simulink model "MPC_mobile_base_KIN_IPOPT_fast"  (R2018b)
settings: Solver=ode4  StartTime=0.0  StopTime=inf  FixedStep=Tsample  RelTol=1e-3
values from neighbouring files (symbols this model uses):
  N = 20    [STEP.m]    (also in ZZ_MIO_STEP.m = 8)
  T = 0.2    [STEP.m]    (also in ZZ_MIO_STEP.m)
  Tsample = 0.01    [STEP.m]    (also in ZZ_MIO_STEP.m)
  xd = [linspace(0,5,length(tt));0.5*ones(size(tt));zeros(size(tt))]    [STEP.m]    (also in ZZ_MIO_STEP.m = [linspace(0,5,length(tt));0.25*ones(size(tt));zeros(size(tt))
undefined symbols (not defined in the file or in its folder): DiscIntNeverNeededParam
libraries: simulink x2, templibrary x1
settings Model: Creator=francesco  LastModifiedBy=francesco

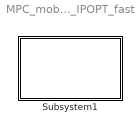
== system MPC_mobile_base_KIN_IPOPT_fast ==
  Subsystem1 : Subsystem  InitFcn=|
      | clearvars -EXCEPT  xd N T Tsample tt
      | 
      | import casadi.*
      | 
      | 
      | %%%%%%%%%%%% SETTINGS %%%%%%%%%%%%%%%%%%%%%
      | 
      | fs = 1/T; % Sampling frequency [hz]
      | m  = 2;
      | T_horizon=(0:N-1)*T;
      | 
      | Ak= diag([100    100    100]);
      | 
      | Vpmax=inf;  %  [m/s^2]
      | Wpmax=3; %  [rad/s^2]
      | 
      | Vpmax=Vpmax*T;
      | Wpmax=Wpmax*T;
      | %%%%%%%%%%%% MODELING %%%%%%%%%%%%%%%%%%%%%
      | x  = MX.sym('x',3);
      | Xd  = MX.sym('Xd',3,N);
      | t  = MX.sym('t');
      | x0 = MX.sym('x0',3);
      | U0  = MX.sym('U0',2,1);
      | 
      | p = MX.sym('p',8);
      | 
      | % xdot = [(p(1)*t^2+p(2)*t+p(3))*cos(x(3)); ...
      | %         (p(1)*t^2+p(2)*t+p(3))*sin(x(3)); ...
      | %         (p(4)*t^3+p(5)*t^2+p(6)*t+p(7))         ];
      | 
      | xdot = [(p(1)*t^3+p(2)*t^2+p(3)*t+p(4))*cos(x(3)); ...
      |         (p(1)*t^3+p(2)*t^2+p(3)*t+p(4))*sin(x(3)); ...
      |         (p(5)*t^3+p(6)*t^2+p(7)*t+p(8))         ];
      | 
      | % Form an ode function
      | ode = Function('ode',{x,p,t},{xdot});
      | 
      | %%%%%%%%%%%% Creating a simulator %%%%%%%%%%
      | N_steps_per_sample = 2;
      | dt = 1/fs/N_steps_per_sample;
      | 
      | % Build an integrator for this system: Runge Kutta 4 integrator
      | k1 = ode(x,p,t);
      | k2 = ode(x+dt/2.0*k1,p,t+dt/2.0);
      | k3 = ode(x+dt/2.0*k2,p,t+dt/2.0);
      | k4 = ode(x+dt*k3,p,t+dt/2.0);
      | 
      | xstep = x+dt/6.0*(k1+2*k2+2*k3+k4);
      | 
      | % Create a function that simulates one step propagation in a sample
      | one_step = Function('one_step',{x, p, t},{xstep});
      | 
      | X = x;
      | for i=1:N_steps_per_sample
      |     X = one_step(X, p, t);
      | end
      | 
      | % Create a function that simulates all step propagation on a sample
      | one_sample = Function('one_sample',{x, p, t}, {X});
      | 
      | % speedup trick: expand into scalar operations
      | one_sample = one_sample.expand();
      | 
      | 
      | %%%%%%%%%%%% Simulating the system %%%%%%%%%%
      | 
      | all_samples = one_sample.mapaccum('all_samples', N);
      | 
      | %%%%%%%%%%%% Identifying the simulated system: single shooting strategy %%%%%%%%%%
      | 
      | % Note, it is in general a good idea to scale your decision variables such
      | % that they are in the order of ~0.1..100
      | X_forecast = [all_samples(x0, repmat(p,1,N),T_horizon)];
      | 
      | usym = [p(1)*t^3+p(2)*t^2+p(3)*t+p(4); ...
      |         p(5)*t^3+p(6)*t^2+p(7)*t+p(8)];
      |     
      | Usym=Function('Usym',{p,t},{usym});
      | 
      | J=0;
      | g={};
      | lbg=[];
      | ubg=[];
      | 
      | for i=1:N
      | 
      | ex=(X_forecast(1,i)-Xd(1,i));
      | ey=(X_forecast(2,i)-Xd(2,i));
      | eth=(X_forecast(3,i)-Xd(3,i));
      |     
      | J = J + ((i/N)^m)*abs([ex ey eth]*Ak*[ex ey eth].');
      | 
      | if i==1
      |     
      | g = {g{:}, Usym(p,T_horizon(i))-U0 };
      | 
      | else
      |     
      | g = {g{:}, Usym(p,T_horizon(i))-Usym(p,T_horizon(i-1)) };
      | 
      | end
      | 
      | lbg = [lbg; [-Vpmax -Wpmax].'];
      | ubg = [ubg; [ Vpmax  Wpmax].'];
      | 
      | end
      | 
      | Gfunction=Function('Gfunction',{p,U0}, {vertcat(g{:})});
      | 
      | Costfunction=Function('Costfunction',{Xd,p,x0}, {J});
      | 
      | % nlp = struct('x', p, 'f', Costfunction(xd_val,p));%, 'g', G);
      | % solver = nlpsol('solver','ipopt', nlp);
      | % 
      | % 
      | % sol = solver('x0',p0);

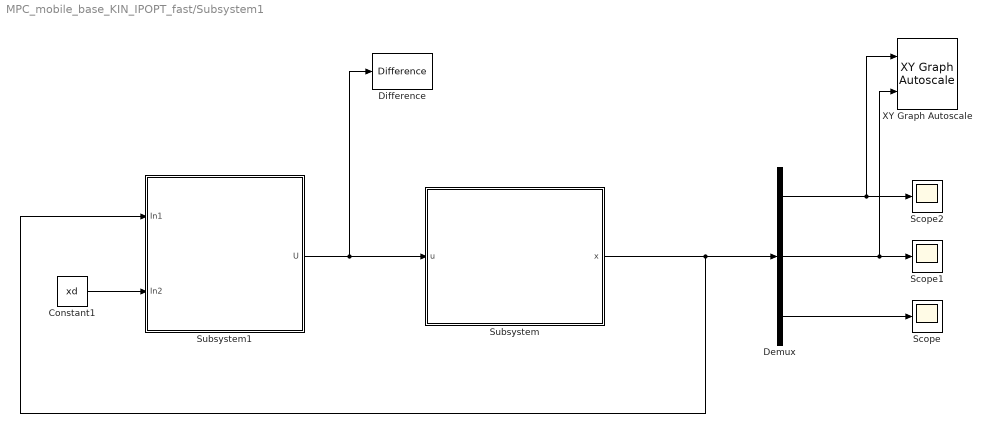
== system MPC_mobile_base_KIN_IPOPT_fast/Subsystem1 ==
  Constant1 : Constant  Value=xd
  Demux : Demux  Outputs=3
  Difference : simulink/Discrete/Difference  ICPrevInput=0.0  OutMin=[]  OutMax=[]  OutDataType=fixdt(1, 16)  OutScaling=2^-10  DoSatur=off
  Scope : Scope
  Scope1 : Scope
  Scope2 : Scope
  Subsystem : Subsystem
      mask Display: disp('{\bf\fontsize{10}KINEMATIC SYSTEM}', 'texmode','on');
  Subsystem1 : Subsystem
  XY Graph Autoscale : templibrary/XY Graph  Autoscale  xmin=-1  xmax=1  ymin=-1  ymax=1  st=-1
  wires:
  Subsystem/1(x) -> Demux/1, Subsystem1/1(In1)
  Demux/1 -> XY Graph Autoscale/1, Scope2/1
  Demux/3 -> Scope/1
  Demux/2 -> XY Graph Autoscale/2, Scope1/1
  Subsystem1/1(U) -> Difference/1, Subsystem/1(u)
  Constant1/1 -> Subsystem1/2(In2)

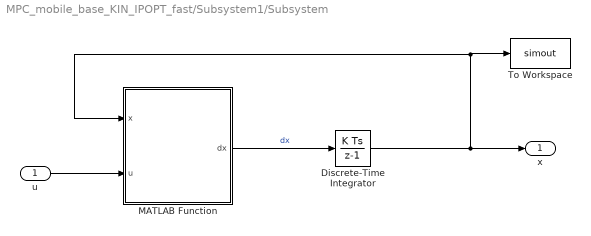
== system MPC_mobile_base_KIN_IPOPT_fast/Subsystem1/Subsystem ==
  u : Inport
  Discrete-Time Integrator : DiscreteIntegrator  InitialCondition=[-0.15 0.1 0]  SampleTime=Tsample  ICPrevOutput=DiscIntNeverNeededParam  ICPrevScaledInput=DiscIntNeverNeededParam
  MATLAB Function : MATLAB Function  TreatAsAtomicUnit=on
  To Workspace : ToWorkspace  VariableName=simout  SaveFormat=Timeseries  SampleTime=T
  x : Outport  SampleTime=Tsample
  wires:
  u/1 -> MATLAB Function/2(u)
  MATLAB Function/1(dx) -> Discrete-Time Integrator/1  "dx"
  Discrete-Time Integrator/1 -> MATLAB Function/1(x), To Workspace/1, x/1

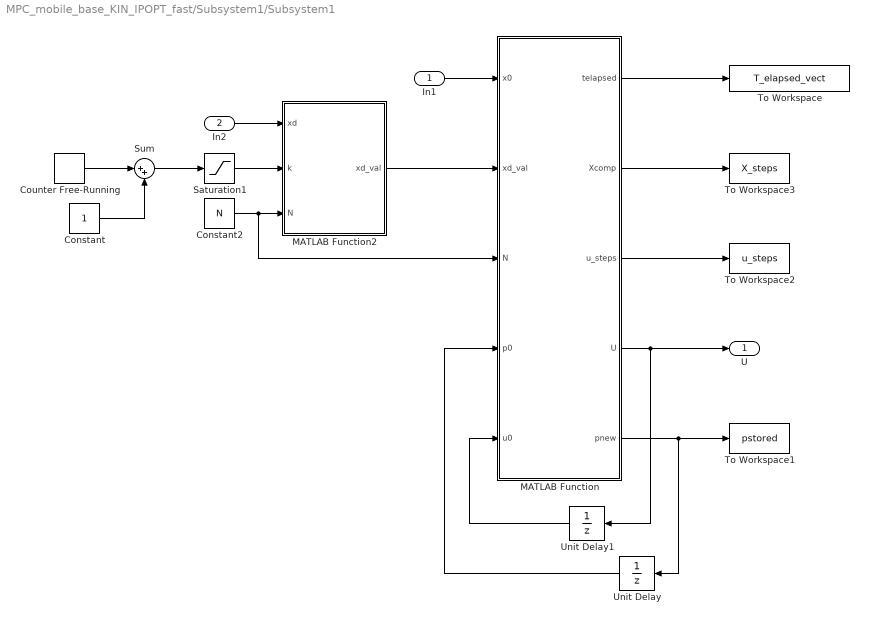
== system MPC_mobile_base_KIN_IPOPT_fast/Subsystem1/Subsystem1 ==
  In1 : Inport
  In2 : Inport  Port=2
  Constant : Constant
  Constant2 : Constant  Value=N
  Counter Free-Running : simulink/Sources/Counter Free-Running  NumBits=12  tsamp=T
  MATLAB Function : MATLAB Function  TreatAsAtomicUnit=on
  MATLAB Function2 : MATLAB Function  TreatAsAtomicUnit=on
  Saturation1 : Saturate  UpperLimit=size(xd,2)
  Sum : Sum  Inputs=|++
  To Workspace : ToWorkspace  VariableName=T_elapsed_vect  SampleTime=T
  To Workspace1 : ToWorkspace  VariableName=pstored  SampleTime=-1
  To Workspace2 : ToWorkspace  VariableName=u_steps  SaveFormat=Structure  SampleTime=-1
  To Workspace3 : ToWorkspace  VariableName=X_steps  SaveFormat=Structure  SampleTime=-1
  Unit Delay : UnitDelay  InitialCondition=[0 0 0 0.1 0 0 0 0].'  SampleTime=T
  Unit Delay1 : UnitDelay  InitialCondition=[0 0].'  SampleTime=T
  U : Outport
  wires:
  Counter Free-Running/1 -> Sum/1
  MATLAB Function/5(pnew) -> To Workspace1/1, Unit Delay/1
  Sum/1 -> Saturation1/1
  Constant/1 -> Sum/2
  In1/1 -> MATLAB Function/1(x0)
  Constant2/1 -> MATLAB Function/3(N), MATLAB Function2/3(N)
  In2/1 -> MATLAB Function2/1(xd)
  MATLAB Function/4(U) -> Unit Delay1/1, U/1
  Unit Delay/1 -> MATLAB Function/4(p0)
  Saturation1/1 -> MATLAB Function2/2(k)
  MATLAB Function2/1(xd_val) -> MATLAB Function/2(xd_val)
  MATLAB Function/1(telapsed) -> To Workspace/1
  Unit Delay1/1 -> MATLAB Function/5(u0)
  MATLAB Function/3(u_steps) -> To Workspace2/1
  MATLAB Function/2(Xcomp) -> To Workspace3/1

== matlab function MPC_mobile_base_KIN_IPOPT_fast/Subsystem1/Subsystem1/MATLAB Function ==
  settings: updateMethod=DISCRETE  sampleTime=T
  data: telapsed output; Xcomp output size=[3,N+1]; u_steps output size=[3,N]; U output; x0 input; pnew output; xd_val input; N input; p0 input; u0 input
function [telapsed,Xcomp,u_steps,U,pnew] = fnc(x0,xd_val,N,p0,u0)

telapsed=0;
u_steps=zeros(2,N);

coder.extrinsic('solver_NLP');

pnew=zeros(8,1);
U=zeros(2,1);
Xcomp=zeros(3,N);

[pnew, U, u_steps, Xcomp, telapsed] = solver_NLP(xd_val,p0,x0,u0);


end

== matlab function MPC_mobile_base_KIN_IPOPT_fast/Subsystem1/Subsystem1/MATLAB Function2 ==
  settings: updateMethod=DISCRETE  sampleTime=T
  data: xd input; k input; N input; xd_val output size=[3,N]
function xd_val = fcn(xd,k,N)

xd_val=zeros(3,N);

if size(xd,2)-k>N-1
h=xd(:,k+1:k+N);
      
else
h=[xd(:,k+1:end) xd(:,end)*ones(1,N-(size(xd,2)-k))];

end
xd_val = h;

end

== matlab function MPC_mobile_base_KIN_IPOPT_fast/Subsystem1/Subsystem/MATLAB Function ==
  settings: updateMethod=DISCRETE  sampleTime=Tsample
  data: x input; dx output; u input size=[2 1]
function dx = sys_dynamics(x,u)
dx=zeros(1,3);
dx(1,1)=u(1,1)*cos(x(3));
dx(1,2)=u(1,1)*sin(x(3));
dx(1,3)=u(2,1);

end
